simulink model "pid_V03"  (R2024b)
settings: Solver=VariableStepAuto  StartTime=0.0  StopTime=40  RelTol=1e-3
undefined symbols (not defined in the file or in its folder): omega_0, p0, R0, v0
settings Model: Creator=bojack  LastModifiedBy=bojack

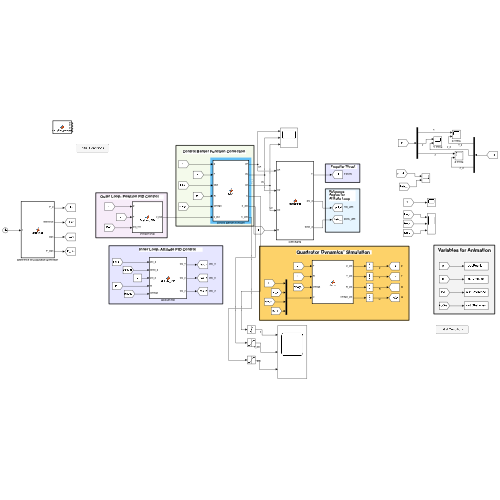
[thumbnail: Simulink's stored preview of the top-level diagram]
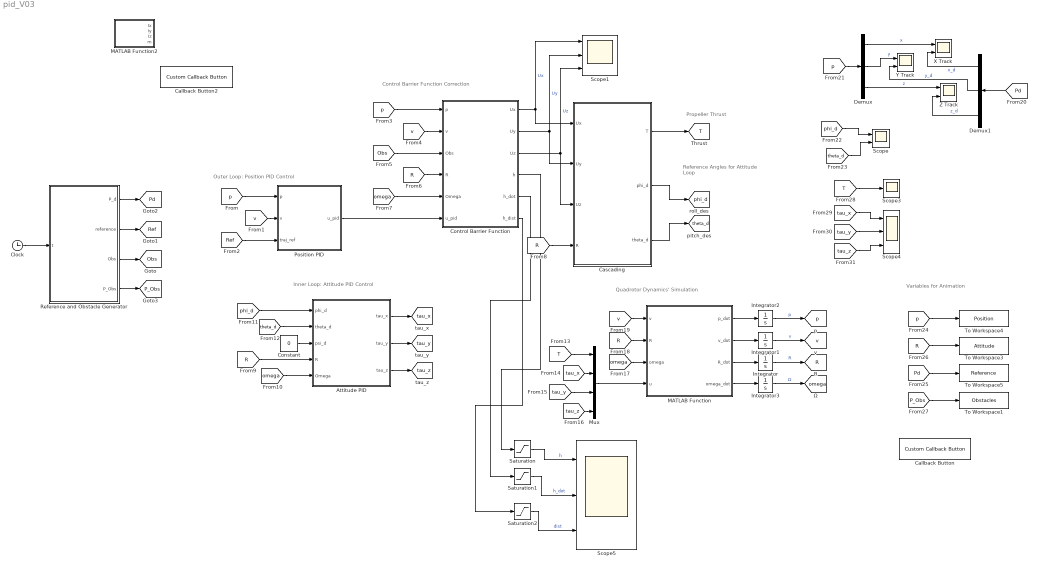
== system pid_V03 ==
  note: Inner Loop: Attitude PID Control
  note: Outer Loop: Position PID Control
  note: Control Barrier Function Correction
  note: Reference Angles for
      | Attitude Loop
  note: Propeller Thrust
  note: Quadrotor Dynamics' Simulation
  note: Variables for Animation
  Attitude PID : MATLAB Function
  Callback Button : CustomCallbackButton  Configuration="{\"components\":[{\"name\":\"BackgroundImageComponent\",\"settings\":{\"image\":{\"size\":[0,0],\"src\":\"default\",\"srcOrientation\":\"Right\"},\"position\":[0,0,1,1]}},{\"name\":\"ButtonStateComponent\",\"settings\":{\"buttonType\":\"momentary\",\"clickFcn\":\"p0 = [10 0 0]';\\nv0 = [-0.5 4.5 1]';\\nR0 = eye(3);\\n\\nomega_0 = [0 0 0]';\",\"onValue\":1,\"position\":[0,0,1,1],\"pressDelay\":\"500\",\"pressFcn\":\"\",\"repeatInterval\":\"0\",\"states\":[{\"horizontalAlignment\":\"center\",\"image\":{\"position\":[0,0,1,1],\"size\":[1,1],\"src\":\"default\",\"srcOrientation\":\"Right\"},\"label\":{\"color\":[0.01176470588,0.01176470588,0.01176470588,1],\"icon\":{\"size\":[0,0],\"src\":\"default\",\"srcOrientation\":\"Right\"},\"iconOffset\":0,\"iconPlacement\":\"left\",\"opacity\":1,\"show\":true,\"text\":{\"content\":\"Initial Conditions\",\"font\":\"Helvetica\"}},\"labelOffset\":[0,0],\"verticalAlignment\":\"middle\"},{\"horizontalAlignment\":\"center\",\"image\":{\"position\":[0,0,1,1],\"size\":[1,1],\"src\":\"default\",\"srcOrientation\":\"Right\"},\"label\":{\"color\":[0.01176470588,0.01176470588,0.01176470588,1],\"icon\":{\"size\":[0,0],\"src\":\"default\",\"srcOrientation\":\"Right\"},\"iconOffset\":0,\"iconPlacement\":\"left\",\"opacity\":1,\"show\":true,\"text\":{\"content\":\"Initial Conditions\",\"font\":\"Helvetica\"}},\"labelOffset\":[0,0],\"verticalAlignment\":\"middle\"},{\"horizontalAlignment\":\"center\",\"image\":{\"position\":[0,0,1,1],\"size\":[1,1],\"src\":\"default\",\"srcOrientation\":\"Right\"},\"label\":{\"color\":[0.01176470588,0.01176470588,0.01176470588,1],\"icon\":{\"size\":[0,0],\"src\":\"default\",\"srcOrientation\":\"Right\"},\"iconOffset\":0,\"iconPlacement\":\"left\",\"opacity\":1,\"show\":true,\"text\":{\"content\":\"Initial Conditions\",\"font\":\"Helvetica\"}},\"labelOffset\":[0,0],\"verticalAlignment\":\"middle\"},{\"horizontalAlignment\":\"center\",\"image\":{\"position\":[0,0,1,1],\"size\":[1,1],\"src\":\"default\",\"srcOrientation\":\"Right\"},\"label\":{\"color\":[0.01176470588,0.01176470588,0.01176470588,1],\"icon\":{\"size\":[0,0],\"src\":\"default\",\"srcOrientation\":\"Right\"},\"iconOffset\":0,\"iconPlacement\":\"left\",\"opacity\":1,\"show\":true,\"text\":{\"content\":\"Initial Conditions\",\"font\":\"Helvetica\"}},\"labelOffset\":[0,0],\"verticalAlignment\":\"middle\"}]}},{\"name\":\"ForegroundImageComponent\",\"settings\":{\"image\":{\"size\":[0,0],\"src\":\"default\",\"srcOrientation\":\"Right\"},\"isForeground\":1,\"position\":[0,0,1,1]}}],\"settings\":{\"BindingType\":\"standalone\",\"backgroundColor\":[244,244,244,1],\"backgroundOffset\":0.2,\"backgroundOpacity\":1,\"fixedAspectRatio\":\"off\",\"foregroundColor\":[0.01176470588,0.01176470588,0.01176470588,1],\"migratedFromLegacy\":true,\"useBackgroundColor\":true,\"variant\":\"callback\",\"version\":\"R2023a\"},\"type\":\"Button\"}"  CustomBackgroundColor="{\"color\":[0.9568627450980393,0.9568627450980393,0.9568627450980393],\"show\":true}"
  Callback Button2 : CustomCallbackButton  Configuration="{\"components\":[{\"name\":\"BackgroundImageComponent\",\"settings\":{\"image\":{\"size\":[0,0],\"src\":\"default\",\"srcOrientation\":\"Right\"},\"position\":[0,0,1,1]}},{\"name\":\"ButtonStateComponent\",\"settings\":{\"buttonType\":\"momentary\",\"clickFcn\":\"p0 = [10 0 0]';\\nv0 = [-0.5 4.5 1]';\\nR0 = eye(3);\\n\\nomega_0 = [0 0 0]';\",\"onValue\":1,\"position\":[0,0,1,1],\"pressDelay\":\"500\",\"pressFcn\":\"\",\"repeatInterval\":\"0\",\"states\":[{\"horizontalAlignment\":\"center\",\"image\":{\"position\":[0,0,1,1],\"size\":[1,1],\"src\":\"default\",\"srcOrientation\":\"Right\"},\"label\":{\"color\":[0.01176470588,0.01176470588,0.01176470588,1],\"icon\":{\"size\":[0,0],\"src\":\"default\",\"srcOrientation\":\"Right\"},\"iconOffset\":0,\"iconPlacement\":\"left\",\"opacity\":1,\"show\":true,\"text\":{\"content\":\"Initial Conditions\",\"font\":\"Helvetica\"}},\"labelOffset\":[0,0],\"verticalAlignment\":\"middle\"},{\"horizontalAlignment\":\"center\",\"image\":{\"position\":[0,0,1,1],\"size\":[1,1],\"src\":\"default\",\"srcOrientation\":\"Right\"},\"label\":{\"color\":[0.01176470588,0.01176470588,0.01176470588,1],\"icon\":{\"size\":[0,0],\"src\":\"default\",\"srcOrientation\":\"Right\"},\"iconOffset\":0,\"iconPlacement\":\"left\",\"opacity\":1,\"show\":true,\"text\":{\"content\":\"Initial Conditions\",\"font\":\"Helvetica\"}},\"labelOffset\":[0,0],\"verticalAlignment\":\"middle\"},{\"horizontalAlignment\":\"center\",\"image\":{\"position\":[0,0,1,1],\"size\":[1,1],\"src\":\"default\",\"srcOrientation\":\"Right\"},\"label\":{\"color\":[0.01176470588,0.01176470588,0.01176470588,1],\"icon\":{\"size\":[0,0],\"src\":\"default\",\"srcOrientation\":\"Right\"},\"iconOffset\":0,\"iconPlacement\":\"left\",\"opacity\":1,\"show\":true,\"text\":{\"content\":\"Initial Conditions\",\"font\":\"Helvetica\"}},\"labelOffset\":[0,0],\"verticalAlignment\":\"middle\"},{\"horizontalAlignment\":\"center\",\"image\":{\"position\":[0,0,1,1],\"size\":[1,1],\"src\":\"default\",\"srcOrientation\":\"Right\"},\"label\":{\"color\":[0.01176470588,0.01176470588,0.01176470588,1],\"icon\":{\"size\":[0,0],\"src\":\"default\",\"srcOrientation\":\"Right\"},\"iconOffset\":0,\"iconPlacement\":\"left\",\"opacity\":1,\"show\":true,\"text\":{\"content\":\"Initial Conditions\",\"font\":\"Helvetica\"}},\"labelOffset\":[0,0],\"verticalAlignment\":\"middle\"}]}},{\"name\":\"ForegroundImageComponent\",\"settings\":{\"image\":{\"size\":[0,0],\"src\":\"default\",\"srcOrientation\":\"Right\"},\"isForeground\":1,\"position\":[0,0,1,1]}}],\"settings\":{\"BindingType\":\"standalone\",\"backgroundColor\":[244,244,244,1],\"backgroundOffset\":0.2,\"backgroundOpacity\":1,\"fixedAspectRatio\":\"off\",\"foregroundColor\":[0.01176470588,0.01176470588,0.01176470588,1],\"migratedFromLegacy\":true,\"useBackgroundColor\":true,\"variant\":\"callback\",\"version\":\"R2023a\"},\"type\":\"Button\"}"  CustomBackgroundColor="{\"color\":[0.9568627450980393,0.9568627450980393,0.9568627450980393],\"show\":true}"
  Cascading : MATLAB Function  TreatAsAtomicUnit=on
  Clock : Clock
  Constant : Constant  Value=0
  Control Barrier Function : MATLAB Function  TreatAsAtomicUnit=on
  Demux : Demux  Outputs=3
  Demux1 : Demux  Outputs=3
  Integrator : Integrator  InitialCondition=R0
  Integrator1 : Integrator  InitialCondition=v0
  Integrator2 : Integrator  InitialCondition=p0
  Integrator3 : Integrator  InitialCondition=omega_0
  MATLAB Function : MATLAB Function  TreatAsAtomicUnit=on
  MATLAB Function2 : MATLAB Function  TreatAsAtomicUnit=on
  Mux : Mux
  Position PID : MATLAB Function
  Reference and Obstacle Generator : MATLAB Function  TreatAsAtomicUnit=on
  Saturation : Saturate  UpperLimit=10  LowerLimit=-10
  Saturation1 : Saturate  UpperLimit=10  LowerLimit=-10
  Saturation2 : Saturate  UpperLimit=10  LowerLimit=-10
  Scope : Scope  NumInputPorts=2
  Scope1 : Scope  NumInputPorts=3
  Scope3 : Scope
  Scope4 : Scope  NumInputPorts=3
  Scope5 : Scope  NumInputPorts=3
  To Workspace1 : ToWorkspace  VariableName=Obstacles  SaveFormat=Structure With Time  SampleTime=0.1
  To Workspace3 : ToWorkspace  VariableName=Attitude  SaveFormat=Structure With Time  SampleTime=0.1
  To Workspace4 : ToWorkspace  VariableName=Position  SaveFormat=Structure With Time  SampleTime=0.1
  To Workspace5 : ToWorkspace  VariableName=Reference  SaveFormat=Structure With Time  SampleTime=0.1
  X Track : Scope  NumInputPorts=2
  Y Track : Scope  NumInputPorts=2
  Z Track : Scope  NumInputPorts=2
  tag scope: Obs=global, P_Obs=global, Pd=global, R=global, Ref=global, T=global, omega=global, p=global, phi_d=global, tau_x=global, tau_y=global, tau_z=global, theta_d=global, v=global
  wires:
  Integrator3/1 -> [omega]  "Ω"
  MATLAB Function/4(omega_dot) -> Integrator3/1
  Integrator2/1 -> [p]  "p"
  MATLAB Function/1(p_dot) -> Integrator2/1
  Integrator1/1 -> [v]  "v"
  Integrator/1 -> [R]  "R"
  MATLAB Function/3(R_dot) -> Integrator/1
  MATLAB Function/2(v_dot) -> Integrator1/1
  [p] -> Position PID/1(p)
  [v] -> Position PID/2(v)
  [Ref] -> Position PID/3(traj_ref)
  Position PID/1(u_pid) -> Control Barrier Function/6(u_pid)
  [v] -> Control Barrier Function/2(v)
  [p] -> Control Barrier Function/1(p)
  [Obs] -> Control Barrier Function/3(Obs)
  [R] -> Control Barrier Function/4(R)
  [omega] -> Control Barrier Function/5(Omega)
  Control Barrier Function/2(Uy) -> Cascading/2(Uy), Scope1/2  "Uy"
  Control Barrier Function/3(Uz) -> Cascading/3(Uz), Scope1/3  "Uz"
  Control Barrier Function/1(Ux) -> Cascading/1(Ux), Scope1/1  "Ux"
  [R] -> Cascading/4(R)
  [R] -> Attitude PID/4(R)
  [omega] -> Attitude PID/5(Omega)
  Constant/1 -> Attitude PID/3(psi_d)
  Cascading/1(T) -> [T]
  Cascading/2(phi_d) -> [phi_d]
  Cascading/3(theta_d) -> [theta_d]
  [theta_d] -> Attitude PID/2(theta_d)
  [phi_d] -> Attitude PID/1(phi_d)
  Attitude PID/2(tau_y) -> [tau_y]
  Attitude PID/1(tau_x) -> [tau_x]
  Attitude PID/3(tau_z) -> [tau_z]
  [T] -> Mux/1
  [tau_x] -> Mux/2
  [tau_y] -> Mux/3
  [tau_z] -> Mux/4
  [R] -> MATLAB Function/2(R)
  [omega] -> MATLAB Function/3(omega)
  [v] -> MATLAB Function/1(v)
  Reference and Obstacle Generator/3(Obs) -> [Obs]
  Reference and Obstacle Generator/2(reference) -> [Ref]
  Reference and Obstacle Generator/1(P_d) -> [Pd]
  Clock/1 -> Reference and Obstacle Generator/1(t)
  [p] -> Demux/1
  Demux/1 -> X Track/1  "x"
  Demux/2 -> Y Track/1  "y"
  Demux/3 -> Z Track/1  "z"
  [Pd] -> Demux1/1
  Demux1/1 -> X Track/2  "x_d"
  Demux1/2 -> Y Track/2  "y_d"
  Demux1/3 -> Z Track/2  "z_d"
  [phi_d] -> Scope/1
  [theta_d] -> Scope/2
  Control Barrier Function/4(h) -> Saturation/1
  [p] -> To Workspace4/1
  [R] -> To Workspace3/1
  [Pd] -> To Workspace5/1
  [P_Obs] -> To Workspace1/1
  Reference and Obstacle Generator/4(P_Obs) -> [P_Obs]
  [T] -> Scope3/1
  [tau_x] -> Scope4/1
  [tau_y] -> Scope4/2
  [tau_z] -> Scope4/3
  Mux/1 -> MATLAB Function/4(u)
  Control Barrier Function/5(h_dot) -> Saturation1/1
  Saturation/1 -> Scope5/1  "h"
  Saturation1/1 -> Scope5/2  "h_dot"
  Saturation2/1 -> Scope5/3  "dist"
  Control Barrier Function/6(h_dist) -> Saturation2/1

== matlab function pid_V03/MATLAB Function2 ==
  data: Ix output; Iy output; Iz output; m output
function [Ix, Iy, Iz, m] = crazyflie_params()
J = [16.6e-6, 0.83e-6, 0.72e-6;
      0.83e-6, 16.6e-6, 1.8e-6;
      0.72e-6, 1.8e-6, 29.3e-6];

%% APPROX
Ix = 16.6e-6;
Iy = 16.6e-6;
Iz =  29.3e-6;

m = 0.027; % Kg

== matlab function pid_V03/MATLAB Function ==
  data: v input; p_dot output; v_dot output; R input; R_dot output; omega input; omega_dot output; u input
function [p_dot, v_dot, R_dot, omega_dot]= drone(v,R,omega, u)

% States
wx = omega(1);
wy = omega(2);
wz = omega(3);

% Inputs
T = u(1);
Tau = u(2:4);

% Parameters
Ix = 16.6e-6; % [kg*m^2]
Iy = 16.6e-6;
Iz =  29.3e-6;

J = diag([Ix Iy Iz]);
%J = eye(3)*0.01;%diag([Ix Iy Iz]);
g = 9.81;
m = 0.027;


e3 = [0 0 1]';
S = [0 -wz wy; wz 0 -wx; -wy wx 0];

% Gyroscopic effects
wx_gyro = 0;
wy_gyro = 0;

w_gyro = [wx_gyro wy_gyro 0]';
%% STATE SPACE MODEL
p_dot = v;
v_dot = -e3*g + R*e3*T/m;
R_dot = R*S;
omega_dot = J\(cross(omega,J*omega)+w_gyro+Tau);

== matlab function pid_V03/Position PID ==
  data: p input; v input; u_pid output; traj_ref input
function u_pid  = Position_PID(p, v, traj_ref)
%% Quadrotor model

% Gravity
g = 9.81;   % [ms^-2]

%% PID CONTROLLER PARAMETERS
%
Kx =0.1;    
Kvx = 0.54;

Ky = 0.1;
Kvy = 0.5;

Kz = 2;
Kvz = 3;


Kx = 1.5;    
Kvx = 2.5;

Ky = 1.5;
Kvy = 2.5;

Kz = 1.5;
Kvz = 2.5;

%{
Kx = 0.375;    
Kvx = 1.25;

Ky = 0.375;
Kvy = 1.25;

Kz = 0.375;
Kvz = 1.25;
%}
%% State

% Position
x = p(1);
y = p(2);
z = p(3);

% Velocity
vx = v(1);
vy = v(2);
vz = v(3);


%% _____ Reference _____
P_d = traj_ref(:,1);
dP_d = traj_ref(:,2);
ddP_d = traj_ref(:,3);

x_d = P_d(1);
y_d = P_d(2);
z_d = P_d(3);

vx_d = dP_d(1);
vy_d = dP_d(2);
vz_d = dP_d(3);

ax_d = ddP_d(1);
ay_d = ddP_d(2);
az_d = ddP_d(3);

%% Nominal Position Controller
Ux = Kx*(x_d-x) + Kvx*(vx_d-vx) + ax_d;
Uy = Ky*(y_d-y) + Kvy*(vy_d-vy) + ay_d;
Uz = Kz*(z_d-z) + Kvz*(vz_d-vz) + az_d;

u_pid = [Ux Uy Uz]';

== matlab function pid_V03/Control Barrier Function ==
  data: p input; Ux output; v input; Obs input; R input; Omega input; u_pid input; Uy output; Uz output; h output; h_dot output; h_dist output
function [Ux, Uy, Uz,h, h_dot, h_dist] = CBF(p,v,Obs,R,Omega,u_pid)
%% _____ CBF _____

M = diag([1/2^2 1/2^2 1/1^2]);
delta = 1.0;
r = 2;
mu = 0.02;

%% Obstacles
n_Obs = size(Obs,1)/3;
P_Obs = Obs(1:n_Obs,:)';
dP_Obs = Obs(n_Obs+1:2*n_Obs,:)';
ddP_Obs = Obs(2*n_Obs+1:3*n_Obs,:)';

%% Find Closest Obstacle
D_Matrix = p - P_Obs;
D_vec = diag(D_Matrix'*D_Matrix);

[~, D_index] = min(D_vec);
p_bar = P_Obs(:,D_index);
v_bar = dP_Obs(:,D_index);
a_bar = ddP_Obs(:,D_index);


V = p - p_bar;
V_dot = (v - v_bar);


S = [0 -Omega(3) Omega(2); Omega(3) 0 -Omega(1); -Omega(2) Omega(1) 0];

Q = R'*M*R;
Q = R'*M*R;
Q_dot = Q*S - S*Q;

l = V + mu*V_dot;

h = l'*Q*l;
h_dot = l'*Q_dot*l + 2*l'*Q*(V_dot + mu*u_pid);

alpha = 2*norm(Omega)*max(diag(M))/min(diag(M));
u = 0;
if h > delta || h_dot > 0
u = u_pid;
else
    Proj = Q*l/(l'*Q*Q*l)*l'*Q;
    Proj_perp = eye(3) - Proj;
    u = -Proj/mu*V_dot + Proj_perp*u_pid;
end
%{
Proj = Q*l/(l'*Q*Q*l)*l'*Q;
Proj_perp = eye(3) - Proj;
u = -Proj*V_dot/mu + Proj_perp*u_pid/2;
h_cbf = h_dot + alpha*h;
%}

%{
dir_unom = uNominal/sqrt(uNominal'*uNominal);
dir_u = u/sqrt(u'*u);
direz_u = dir_u'*dir_unom;
%}

% CBF evaluation index
Q  = R'*diag([1/0.5^2 1/0.5^2 1/0.25^2])*R;
h_dist = V'*Q*V - 1;
Ux = u(1);
Uy = u(2);
Uz = u(3);


%{
if abs(Ux) > 50 
    Ux = sign(Ux)*50;
end
if abs(Uy) > 50 
    Uy = sign(Uy)*50;
end
if abs(Uz) > 50 
    Uz = sign(Uz)*50;
end
%}

== matlab function pid_V03/Cascading ==
  data: Ux input; T output; Uy input; Uz input; phi_d output; theta_d output; R input
function [T, phi_d, theta_d] = cascading(Ux,Uy,Uz, R)
% Gravity
g = 9.81;

% Mass
m = 0.027;

% Attitude Euler
eul_angles = rotm2eul(R,'XYZ');
phi = eul_angles(1); 
theta = eul_angles(2);  
psi = eul_angles(3); 

% Thrust Computation
T = (g + Uz)* ( m/( cos(phi)*cos(theta) ));

%desired attitude from desired thrust direction
theta_d = atan2(Ux*cos(psi) + Uy*sin(psi), (Uz+g));
theta_d = rad2deg(theta_d);


if abs(theta_d)>45
    theta_d = 45*sign(theta_d);
end


% Notice cosd for theta_d
phi_d = atan2(cosd(theta_d)*(Ux*sind(psi) - Uy*cos(psi)), (Uz+g));
phi_d = rad2deg(phi_d);


if abs(phi_d)>45
    phi_d = 45*sign(phi_d);
end

== matlab function pid_V03/Attitude PID ==
  data: phi_d input; theta_d input; psi_d input; R input; Omega input; tau_x output; tau_y output; tau_z output
function [tau_x, tau_y, tau_z]  = Attitude_PID(phi_d, theta_d, psi_d, R, Omega)
%% Drone Parameters
Ix = 16.6e-6; % [kg*m^2]
Iy = 16.6e-6;
Iz =  29.3e-6;

%% State
eul_angles = rad2deg(rotm2eul(R, "XYZ"));

phi = eul_angles(1); 
theta = eul_angles(2);  
psi = eul_angles(3); 

wx = rad2deg(Omega(1));
wy = rad2deg(Omega(2));
wz = rad2deg(Omega(3));

%% PID Gains
K_phi = 120;
K_wx = 22;

K_theta = 120;
K_wy = 22;

K_psi = 10*0.1;
K_wz = 10;

tau_x  = Ix*deg2rad((K_phi * (phi_d - phi) + K_wx * -wx));
tau_y  = Iy*deg2rad((K_theta * (theta_d - theta) + K_wy * -wy));
tau_z  = Iz*deg2rad((K_psi * (psi_d - psi) + K_wz * -wz));

== matlab function pid_V03/Reference and Obstacle Generator ==
  data: t input; P_d output; reference output; Obs output; P_Obs output
function [P_d, reference, Obs, P_Obs] = generate(t)
%{
w = 0.5;
R = 10;

x_d = R*cos(w*t);
y_d = R*sin(w*t);
z_d = w*t;

vx_d = -w*R*sin(w*t);
vy_d = w*R*cos(w*t);
vz_d = w;

ax_d = -w^2*R*cos(w*t);
ay_d = -w^2*R*sin(w*t);
az_d = 0;

%%%%  %%%%%%
P_d = [x_d y_d z_d]';
dP_d = [vx_d vy_d vz_d]';
ddP_d = [ax_d ay_d az_d]';

reference = [P_d dP_d ddP_d];

P_Obs = [0 R pi/2+0.2; -R 0 pi+0.2; R 0 2*pi+0.2];
%}
x_d = 1*t;
y_d = 0;
z_d = 0;

vx_d = 1;
vy_d = 0;
vz_d = 0;

ax_d = 0;
ay_d = 0;
az_d = 0;

%%%%  %%%%%%
R = 10;
P_d = [x_d y_d z_d]';
dP_d = [vx_d vy_d vz_d]';
ddP_d = [ax_d ay_d az_d]';

reference = [P_d dP_d ddP_d];

%{
P_Obs = [20 0 -1; %[z x(sotto) y(sinistra]
         20 2 -1;
         19.6 0.4 1;
         20 -1.5 -0.3;
         20 0 3;
         20 1 0;
         20 2 1; 
         20 -2.2 4; %3
         20 -2.2 -1;
         20 -3.5 1.5]; %-4.3
%}

P_Obs = [   20.0000   -3.0000   -1.5000;
   20.0000   -3.0000   -1.2000;
   20.0000   -3.0000   -0.9000;
   20.0000   -3.0000   -0.6000;
   20.0000   -3.0000   -0.3000;
   20.0000   -3.0000         0;
   20.0000   -3.0000    0.3000;
   20.0000   -3.0000    0.6000;
   20.0000   -3.0000    0.9000;
   20.0000   -3.0000    1.2000;
   20.0000   -3.0000    1.5000;
   20.0000   -2.4000   -1.5000;
   20.0000   -2.4000   -1.2000;
   20.0000   -2.4000   -0.9000;
   20.0000   -2.4000   -0.6000;
   20.0000   -2.4000   -0.3000;
   20.0000   -2.4000         0;
   20.0000   -2.4000    0.3000;
   20.0000   -2.4000    0.6000;
   20.0000   -2.4000    0.9000;
   20.0000   -2.4000    1.2000;
   20.0000   -2.4000    1.5000;
   20.0000   -1.8000   -1.5000;
   20.0000   -1.8000   -1.2000;
   20.0000   -1.8000   -0.9000;
   20.0000   -1.8000   -0.6000;
   20.0000   -1.8000   -0.3000;
   20.0000   -1.8000         0;
   20.0000   -1.8000    0.3000;
   20.0000   -1.8000    0.6000;
   20.0000   -1.8000    0.9000;
   20.0000   -1.8000    1.2000;
   20.0000   -1.8000    1.5000;
   20.0000   -1.2000   -1.5000;
   20.0000   -1.2000   -1.2000;
   20.0000   -1.2000   -0.9000;
   20.0000   -1.2000   -0.6000;
   20.0000   -1.2000   -0.3000;
   20.0000   -1.2000         0;
   20.0000   -1.2000    0.3000;
   20.0000   -1.2000    0.6000;
   20.0000   -1.2000    0.9000;
   20.0000   -1.2000    1.2000;
   20.0000   -1.2000    1.5000;
   20.0000   -0.6000   -1.5000;
   20.0000   -0.6000   -1.2000;
   20.0000   -0.6000   -0.9000;
   20.0000   -0.6000   -0.6000;
   20.0000   -0.6000   -0.3000;
   20.0000   -0.6000         0;
   20.0000   -0.6000    0.3000;
   20.0000   -0.6000    0.6000;
   20.0000   -0.6000    0.9000;
   20.0000   -0.6000    1.2000;
   20.0000   -0.6000    1.5000;
   20.0000         0   -1.5000;
   20.0000         0   -1.2000;
   20.0000         0   -0.9000;
   20.0000         0   -0.6000;
   20.0000         0   -0.3000;
   20.0000         0         0;
   20.0000         0    0.3000;
   20.0000         0    0.6000;
   20.0000         0    0.9000;
   20.0000         0    1.2000;
   20.0000         0    1.5000;
   20.0000    0.6000   -1.5000;
   20.0000    0.6000   -1.2000;
   20.0000    0.6000   -0.9000;
   20.0000    0.6000   -0.6000;
   20.0000    0.6000   -0.3000;
   20.0000    0.6000         0;
   20.0000    0.6000    0.3000;
  % 20.0000    0.6000    0.6000;
   20.0000    0.6000    0.9000;
   20.0000    0.6000    1.2000;
   20.0000    0.6000    1.5000;
   20.0000    1.2000   -1.5000;
   20.0000    1.2000   -1.2000;
   20.0000    1.2000   -0.9000;
   20.0000    1.2000   -0.6000;
   20.0000    1.2000   -0.3000;
   20.0000    1.2000         0;
   20.0000    1.2000    0.3000;
  %
   20.0000    1.2000    0.6000;
   20.0000    1.2000    0.9000;
   20.0000    1.2000    1.2000;
   20.0000    1.2000    1.5000;
   20.0000    1.8000   -1.5000;
   20.0000    1.8000   -1.2000;
   20.0000    1.8000   -0.9000;
   20.0000    1.8000   -0.6000;
   20.0000    1.8000   -0.3000;
   20.0000    1.8000         0;
   20.0000    1.8000    0.3000;
   20.0000    1.8000    0.6000;
   20.0000    1.8000    1.2000;
   20.0000    1.8000    1.5000;
   20.0000    2.4000   -1.5000;
   20.0000    2.4000   -1.2000;
   20.0000    2.4000   -0.9000;
   20.0000    2.4000   -0.6000;
   20.0000    2.4000   -0.3000;
   20.0000    2.4000         0;
   20.0000    2.4000    0.3000;
   20.0000    2.4000    0.6000;
   20.0000    2.4000    0.9000;
   20.0000    2.4000    1.2000;
   20.0000    2.4000    1.5000;
   20.0000    3.0000   -1.5000;
   20.0000    3.0000   -1.2000;
   20.0000    3.0000   -0.9000;
   20.0000    3.0000   -0.6000;
   20.0000    3.0000   -0.3000;
   20.0000    3.0000         0;
   20.0000    3.0000    0.3000;
   20.0000    3.0000    0.6000;
   20.0000    3.0000    0.9000;
   20.0000    3.0000    1.2000;
   20.0000    3.0000    1.5000];


dP_Obs = zeros(size(P_Obs,1),3);
ddP_Obs = zeros(size(P_Obs,1),3);

Obs = [P_Obs; dP_Obs; ddP_Obs];
